simulink model "bh_source_XL_bigger"  (R2018a)
settings: Solver=ode4  StartTime=0.0  StopTime=60  FixedStep=0.001  RelTol=1e-5
model workspace (MAT data in the model file):
  Hz = 0.2
  L1x = 0.005
  L1y = 0.75
  L1z = 0.05
  L2x = 0.005
  L2y = 0.5
  L2z = 0.05
  L3x = 0.005
  L3y = 0.25
  L3z = 0.05
  P_mot.Vmax = 12
  P_mot.ID = 0
  P_mot.Ka = 0.04
  P_mot.Ke = 0.04
  P_mot.b = []
  P_mot.I = []
  P_mot.R = 5
  P_mot.L = 0.00063
  P_mot.G = 100
  P_mot.TQ_G_max = 3
  P_mot.TQ_m_max = 0.03
  Rturn = 0.05
  b1_damp = 0.005
  b2_damp = 0.005
  b3_damp = 0.005
  b4_damp = 0.005
  density = 1000
  g = 9.80665
  mass1 = 0.1875
  mass2 = 0.125
  mass3 = 0.0625
  mass4 = 1.57079632679
  theta1_0 = 0
  theta1_dot_0 = 0
  theta2_0 = 0
  theta2_dot_0 = 0
  theta3_0 = 0
  theta3_dot_0 = 0
  theta4_0 = 0
  theta4_dot_0 = 0
libraries: simulink_extras x2
settings Model: Creator=bhorton  LastModifiedBy=bhorton
settings SolverCC: ZeroCrossAlgorithm=Adaptive
settings OptimizationCC: LifeSpan=inf
settings DebuggingCC: SFUnexpectedBacktrackingDiag=warning  SFNoUnconditionalDefaultTransitionDiag=warning  SFExecutionAtInitializationDiag=none
settings CodeAppCC: StateflowObjectComments=on
settings GRTTargetCC: TargetLangStandard=C89/C90 (ANSI)
settings ConfigComp: CovMetricSettings=dw  CovHtmlReporting=on  CovSaveCumulativeToWorkspaceVar=on  CovSaveSingleToWorkspaceVar=on  CovExternalEMLEnable=off
settings SimscapeCC: SimscapeNormalizeSystem=off  SimscapeLogType=all  SimscapeLogDataHistory=10000  SelectedTab=Simscape Multibody
settings ExplorerConfigSet: InternalSimMechanicsExplorerSettings="<ExplorerConfiguration><canonicalview>default</canonicalview><AnimationSetting><BasePlaybackSpeed>1.0</BasePlaybackSpeed><PlaybackSpeedFactor>1.0</PlaybackSpeedFactor></AnimationSetting><TilePanel><TileInfo><Tiles Columns=\"2\" Count=\"4\" Rows=\"2\"><Column Left=\"2\" Weight=\"0.4992\"/><Column Left=\"655\" Weight=\"0.5008\"/><Column Left=\"1310\"/><Row Top=\"2\" Weight=\"0.4984\"/><Row Top=\"475\" Weight=\"0.5016\"/><Row Top=\"950\"/><Tile Height=\"1\" Width=\"1\" X=\"0\" Y=\"0\"/><Tile Height=\"1\" Width=\"1\" X=\"0\" Y=\"1\"/><Tile Height=\"1\" Width=\"1\" X=\"1\" Y=\"0\"/><Tile Height=\"1\" Width=\"1\" X=\"1\" Y=\"1\"/></Tiles></TileInfo><SceneInfo><SceneViewer><BGColor><R>0.60000002384185791</R><G>0.60000002384185791</G><B>0.60000002384185791</B></BGColor><Camera><DoPerspective>off</DoPerspective><Position><X>0.57010570867346566</X><Y>-0.81939487187068383</Y><Z>-0.041325690013103822</Z></Position><Center><X>0.57010570867346566</X><Y>0.37243777720020188</Y><Z>-0.041325690013103822</Z></Center><Up><X>0</X><Y>-0</Y><Z>1</Z></Up><ViewLimDist>1</ViewLimDist><YLim>0.58387397231837834</YLim><XLim>0.8103768064074045</XLim></Camera></SceneViewer><SceneViewer><BGColor><R>0.60000002384185791</R><G>0.60000002384185791</G><B>0.60000002384185791</B></BGColor><Camera><DoPerspective>off</DoPerspective><Position><X>0.51388092361444482</X><Y>0.52196280048326149</Y><Z>0.82022286793681332</Z></Position><Center><X>0.51388092361444482</X><Y>0.52196280048326149</Y><Z>-0.17977713206318668</Z></Center><Up><X>0</X><Y>1</Y><Z>-0</Z></Up><ViewLimDist>1</ViewLimDist><YLim>0.97737746692739225</YLim><XLim>1.3507104907751943</XLim></Camera></SceneViewer><SceneViewer><BGColor><R>0.60000002384185791</R><G>0.60000002384185791</G><B>0.60000002384185791</B></BGColor><Camera><DoPerspective>off</DoPerspective><Position><X>1.5094114010486579</X><Y>0.67796186035410533</Y><Z>-0.0082694811079057073</Z></Position><Center><X>0.47943838776152692</X><Y>0.67796186035410533</Y><Z>-0.0082694811079057073</Z></Center><Up><X>-0</X><Y>0</Y><Z>1</Z></Up><ViewLimDist>1</ViewLimDist><YLim>0.68608550995197048</YLim><XLim>0.95519663670037269</XLim></Camera></SceneViewer><SceneViewer><BGColor><R>0.60000002384185791</R><G>0.60000002384185791</G><B>0.60000002384185791</B></BGColor><Camera><DoPerspective>off</DoPerspective><Position><X>1.2860411296222924</X><Y>0.12259966358168611</Y><Z>0.94383913066063729</Z></Position><Center><X>0.57516484098717713</X><Y>0.83347595221680226</Y><Z>0.23296284202552392</Z></Center><Up><X>-0.40824829046386307</X><Y>0.40824829046386307</Y><Z>0.81649658092772615</Z></Up><ViewLimDist>1</ViewLimDist><YLim>0.94664886749230226</YLim><XLim>1.3123072283262387</XLim></Camera></SceneViewer></SceneInfo></TilePanel><MechEditorPanel><Cameras/><GfxPanelCameraMap/><VideoCreator><PlaybackSpeedRatio>1.0</PlaybackSpeedRatio><FrameRate>30</FrameRate><VideoFormat>Motion JPEG AVI</VideoFormat><FrameSize>auto</FrameSize></VideoCreator></MechEditorPanel></ExplorerConfiguration>"

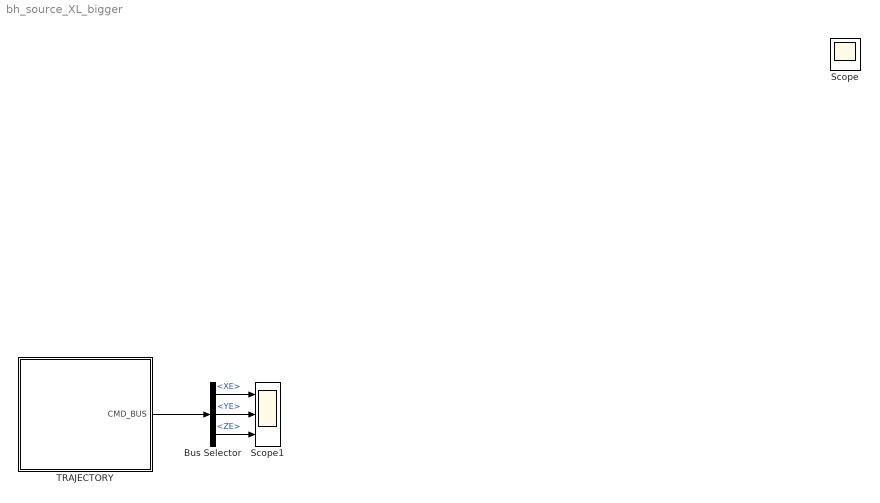
== system bh_source_XL_bigger ==
  Bus Selector : BusSelector  OutputSignals=XYZ_BUS.XE,XYZ_BUS.YE,XYZ_BUS.ZE
  Scope1 : Scope  NumInputPorts=3
  TRAJECTORY : Subsystem
  Scope : Scope
  wires:
  TRAJECTORY/1(CMD_BUS) -> Bus Selector/1
  Bus Selector/1 -> Scope1/1  "<XE>"
  Bus Selector/2 -> Scope1/2  "<YE>"
  Bus Selector/3 -> Scope1/3  "<ZE>"

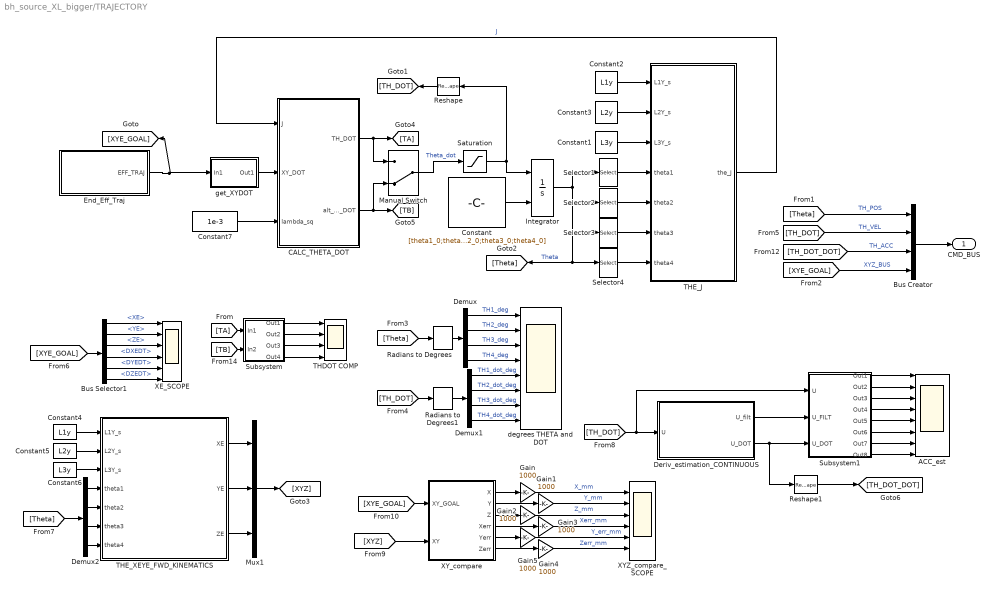
== system bh_source_XL_bigger/TRAJECTORY ==
  ACC_est : Scope  NumInputPorts=8
  Bus Creator : BusCreator  Inputs=4
  Bus Selector1 : BusSelector  OutputSignals=XE,YE,ZE,DXEDT,DYEDT,DZEDT
  CALC_THETA_DOT : MATLAB Function  TreatAsAtomicUnit=on
  Constant : Constant  Value=[theta1_0;theta2_0;theta3_0;theta4_0]  VectorParams1D=off
  Constant1 : Constant  Value=L3y
  Constant2 : Constant  Value=L1y
  Constant3 : Constant  Value=L2y
  Constant4 : Constant  Value=L1y
  Constant5 : Constant  Value=L2y
  Constant6 : Constant  Value=L3y
  Constant7 : Constant  Value=1e-3
  Demux : Demux
  Demux1 : Demux
  Demux2 : Demux
  Deriv_estimation_CONTINUOUS : Subsystem  mask(Derivative Estimation){wn=2*pi*100, p=1, x0_val=0, v0_val=0}
      mask prompts: wn "Natural frequency, wn (rad/sec)"; p "Damping ratio, p"; x0_val "X_IC"; v0_val "X_DOT_IC"
      mask help:
      | A simple derivative estimator using a 2nd order representation between input and output.
      |
      | The integrators use a discrete FORWARd Euler rule, and a sample time needs to be specified.
      mask init:
      | str0 = sprintf('fn = %.2f [Hz]', (wn/(2*pi)));
      | str1 = sprintf('wn = %.2f', wn);
      | str2 = sprintf('p  = %.3g', p);
      | %str3 = sprintf('dt = %.2g', dt);
      | str = char(str0,str1,str2);
      mask Display: disp(str)
  End_Eff_Traj : Subsystem
  Gain{,1..5} (6 alike) : Gain  Gain=1000
  Integrator : Integrator  InitialConditionSource=external
  Manual Switch : ManualSwitch  CurrentSetting=0
  Mux1 : Mux  Inputs=3
  Radians to Degrees : simulink_extras/Transformations/Radians to Degrees
  Radians to Degrees1 : simulink_extras/Transformations/Radians to Degrees
  Reshape : Reshape  OutputDimensionality=Column vector (2-D)
  Reshape1 : Reshape  OutputDimensionality=Column vector (2-D)
  Saturation : Saturate  UpperLimit=6  LowerLimit=-6
  Selector1 : Selector  InputPortWidth=4  IndexOptions=Index vector (dialog)  Indices=1  OutputSizes=1
  Selector2 : Selector  InputPortWidth=4  IndexOptions=Index vector (dialog)  Indices=2  OutputSizes=1
  Selector3 : Selector  InputPortWidth=4  IndexOptions=Index vector (dialog)  Indices=3  OutputSizes=1
  Selector4 : Selector  InputPortWidth=4  IndexOptions=Index vector (dialog)  Indices=4  OutputSizes=1
  Subsystem : Subsystem
  Subsystem1 : Subsystem
  THDOT COMP : Scope  NumInputPorts=4
  THE_J : MATLAB Function  TreatAsAtomicUnit=on
  THE_XEYE_FWD_KINEMATICS : MATLAB Function  TreatAsAtomicUnit=on
  XE_SCOPE : Scope  NumInputPorts=6
  XYZ_compare_SCOPE : Scope  NumInputPorts=6
  XY_compare : Subsystem
  degrees THETA and DOT : Scope  NumInputPorts=8
  get_XYDOT : Subsystem
  CMD_BUS : Outport
  wires:
  Bus Selector1/1 -> XE_SCOPE/1  "<XE>"
  Bus Selector1/2 -> XE_SCOPE/2  "<YE>"
  Bus Selector1/3 -> XE_SCOPE/3  "<ZE>"
  Bus Selector1/4 -> XE_SCOPE/4  "<DXEDT>"
  Bus Selector1/5 -> XE_SCOPE/5  "<DYEDT>"
  Bus Selector1/6 -> XE_SCOPE/6  "<DZEDT>"
  [XYE_GOAL] -> Bus Selector1/1
  Constant/1 -> Integrator/2
  THE_J/1(the_J) -> CALC_THETA_DOT/1(J)  "J"
  get_XYDOT/1(Out1) -> CALC_THETA_DOT/2(XY_DOT)
  Manual Switch/1 -> Saturation/1  "Theta_dot"
  Integrator/1 -> Selector4/1, [Theta], Selector3/1, Selector2/1, Selector1/1  "Theta"
  End_Eff_Traj/1(EFF_TRAJ) -> get_XYDOT/1(In1), [XYE_GOAL]
  Saturation/1 -> Integrator/1, Reshape/1
  Selector4/1 -> THE_J/7(theta4)
  Selector3/1 -> THE_J/6(theta3)
  Selector2/1 -> THE_J/5(theta2)
  Selector1/1 -> THE_J/4(theta1)
  Constant2/1 -> THE_J/1(L1Y_s)
  Constant3/1 -> THE_J/2(L2Y_s)
  Constant1/1 -> THE_J/3(L3Y_s)
  CALC_THETA_DOT/1(TH_DOT) -> [TA], Manual Switch/1
  CALC_THETA_DOT/2(alt_TH_DOT) -> [TB], Manual Switch/2
  Constant7/1 -> CALC_THETA_DOT/3(lambda_sq)
  [TB] -> Subsystem/2(In2)
  [TA] -> Subsystem/1(In1)
  Subsystem/1(Out1) -> THDOT COMP/1
  Subsystem/2(Out2) -> THDOT COMP/2
  Subsystem/3(Out3) -> THDOT COMP/3
  Subsystem/4(Out4) -> THDOT COMP/4
  [TH_DOT] -> Bus Creator/2  "TH_VEL"
  [Theta] -> Bus Creator/1  "TH_POS"
  Bus Creator/1 -> CMD_BUS/1
  Reshape/1 -> [TH_DOT]
  [XYE_GOAL] -> Bus Creator/4  "XYZ_BUS"
  Demux/4 -> degrees THETA and DOT/4  "TH4_deg"
  Demux/3 -> degrees THETA and DOT/3  "TH3_deg"
  Demux/2 -> degrees THETA and DOT/2  "TH2_deg"
  Demux/1 -> degrees THETA and DOT/1  "TH1_deg"
  Demux1/1 -> degrees THETA and DOT/5  "TH1_dot_deg"
  Demux1/2 -> degrees THETA and DOT/6  "TH2_dot_deg"
  Demux1/3 -> degrees THETA and DOT/7  "TH3_dot_deg"
  Demux1/4 -> degrees THETA and DOT/8  "TH4_dot_deg"
  [Theta] -> Radians to Degrees/1
  Radians to Degrees/1 -> Demux/1
  [TH_DOT] -> Radians to Degrees1/1
  Radians to Degrees1/1 -> Demux1/1
  Constant4/1 -> THE_XEYE_FWD_KINEMATICS/1(L1Y_s)
  Constant6/1 -> THE_XEYE_FWD_KINEMATICS/3(L3Y_s)
  Constant5/1 -> THE_XEYE_FWD_KINEMATICS/2(L2Y_s)
  Demux2/1 -> THE_XEYE_FWD_KINEMATICS/4(theta1)
  Demux2/2 -> THE_XEYE_FWD_KINEMATICS/5(theta2)
  Demux2/3 -> THE_XEYE_FWD_KINEMATICS/6(theta3)
  Demux2/4 -> THE_XEYE_FWD_KINEMATICS/7(theta4)
  [Theta] -> Demux2/1
  THE_XEYE_FWD_KINEMATICS/1(XE) -> Mux1/1
  THE_XEYE_FWD_KINEMATICS/3(ZE) -> Mux1/3
  THE_XEYE_FWD_KINEMATICS/2(YE) -> Mux1/2
  Mux1/1 -> [XYZ]
  [TH_DOT] -> Subsystem1/1(U), Deriv_estimation_CONTINUOUS/1(U)
  Subsystem1/1(Out1) -> ACC_est/1
  Subsystem1/2(Out2) -> ACC_est/2
  Subsystem1/3(Out3) -> ACC_est/3
  Subsystem1/4(Out4) -> ACC_est/4
  Subsystem1/5(Out5) -> ACC_est/5
  Subsystem1/6(Out6) -> ACC_est/6
  Subsystem1/7(Out7) -> ACC_est/7
  Subsystem1/8(Out8) -> ACC_est/8
  Deriv_estimation_CONTINUOUS/1(U_filt) -> Subsystem1/2(U_FILT)
  Deriv_estimation_CONTINUOUS/2(U_DOT) -> Reshape1/1, Subsystem1/3(U_DOT)
  [TH_DOT_DOT] -> Bus Creator/3  "TH_ACC"
  Reshape1/1 -> [TH_DOT_DOT]
  [XYZ] -> XY_compare/2(XY)
  [XYE_GOAL] -> XY_compare/1(XY_GOAL)
  Gain/1 -> XYZ_compare_SCOPE/1  "X_mm"
  Gain1/1 -> XYZ_compare_SCOPE/2  "Y_mm"
  Gain2/1 -> XYZ_compare_SCOPE/3  "Z_mm"
  XY_compare/1(X) -> Gain/1
  XY_compare/2(Y) -> Gain1/1
  XY_compare/3(Z) -> Gain2/1
  Gain4/1 -> XYZ_compare_SCOPE/6  "Zerr_mm"
  XY_compare/6(Zerr) -> Gain4/1
  XY_compare/5(Yerr) -> Gain5/1
  Gain5/1 -> XYZ_compare_SCOPE/5  "Y_err_mm"
  Gain3/1 -> XYZ_compare_SCOPE/4  "Xerr_mm"
  XY_compare/4(Xerr) -> Gain3/1

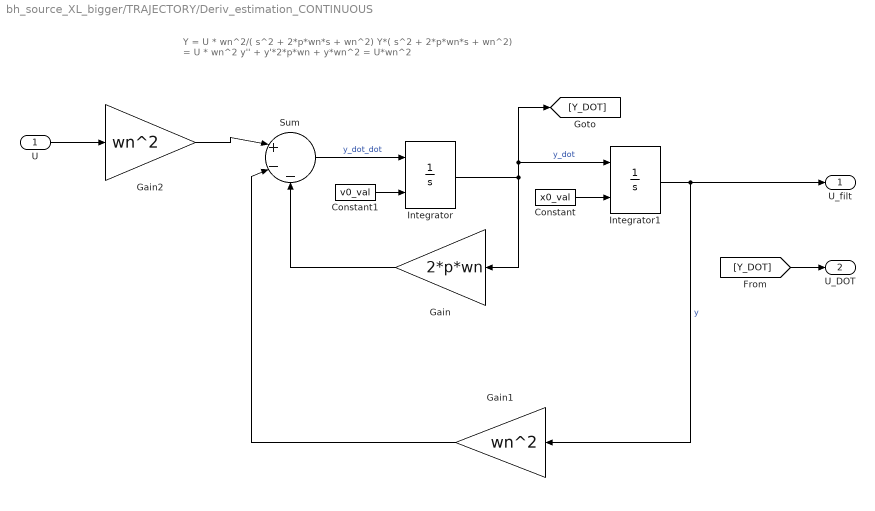
== system bh_source_XL_bigger/TRAJECTORY/Deriv_estimation_CONTINUOUS ==
  note: Y = U *     wn^2/( s^2 + 2*p*wn*s + wn^2)
      | Y*( s^2 + 2*p*wn*s + wn^2) = U * wn^2
      |
      | y'' + y'*2*p*wn + y*wn^2 = U*wn^2
  U : Inport
  Constant : Constant  Value=x0_val
  Constant1 : Constant  Value=v0_val
  Gain : Gain  Gain=2*p*wn
  Gain1 : Gain  Gain=wn^2
  Gain2 : Gain  Gain=wn^2
  Integrator : Integrator  InitialConditionSource=external
  Integrator1 : Integrator  InitialConditionSource=external
  Sum : Sum  Inputs=|+--
  U_filt : Outport
  U_DOT : Outport  Port=2
  wires:
  Integrator/1 -> Integrator1/1, [Y_DOT], Gain/1  "y_dot"
  Sum/1 -> Integrator/1  "y_dot_dot"
  Integrator1/1 -> U_filt/1, Gain1/1  "y"
  U/1 -> Gain2/1
  Gain2/1 -> Sum/1
  Gain/1 -> Sum/3
  Gain1/1 -> Sum/2
  [Y_DOT] -> U_DOT/1
  Constant/1 -> Integrator1/2
  Constant1/1 -> Integrator/2

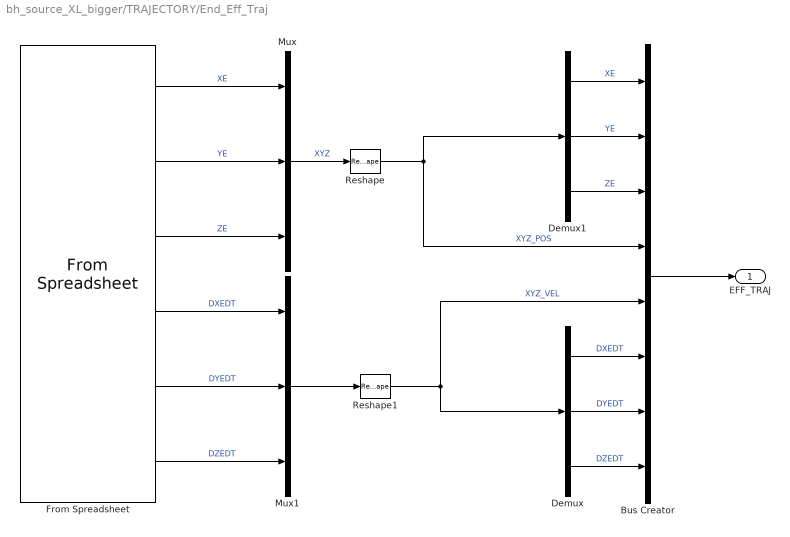
== system bh_source_XL_bigger/TRAJECTORY/End_Eff_Traj ==
  Bus Creator : BusCreator  Inputs=8
  Demux : Demux  Outputs=3
  Demux1 : Demux  Outputs=3
  From Spreadsheet : FromSpreadsheet  FileName=bh_hello_complete.xlsx  SheetName=COMP_SPLINE _4dof  SampleTime=0.001  ExtrapolationBeforeFirstDataPoint=Hold first value  ExtrapolationAfterLastDataPoint=Hold last value
  Mux : Mux  Inputs=3
  Mux1 : Mux  Inputs=3
  Reshape : Reshape  OutputDimensionality=Column vector (2-D)
  Reshape1 : Reshape  OutputDimensionality=Column vector (2-D)
  EFF_TRAJ : Outport
  wires:
  From Spreadsheet/2 -> Mux/2  "YE"
  From Spreadsheet/3 -> Mux/3  "ZE"
  From Spreadsheet/1 -> Mux/1  "XE"
  From Spreadsheet/4 -> Mux1/1  "DXEDT"
  Bus Creator/1 -> EFF_TRAJ/1
  From Spreadsheet/6 -> Mux1/3  "DZEDT"
  From Spreadsheet/5 -> Mux1/2  "DYEDT"
  Demux/1 -> Bus Creator/6  "DXEDT"
  Demux/2 -> Bus Creator/7  "DYEDT"
  Demux/3 -> Bus Creator/8  "DZEDT"
  Demux1/1 -> Bus Creator/1  "XE"
  Demux1/2 -> Bus Creator/2  "YE"
  Demux1/3 -> Bus Creator/3  "ZE"
  Mux/1 -> Reshape/1  "XYZ"
  Mux1/1 -> Reshape1/1
  Reshape/1 -> Bus Creator/4, Demux1/1  "XYZ_POS"
  Reshape1/1 -> Demux/1, Bus Creator/5  "XYZ_VEL"

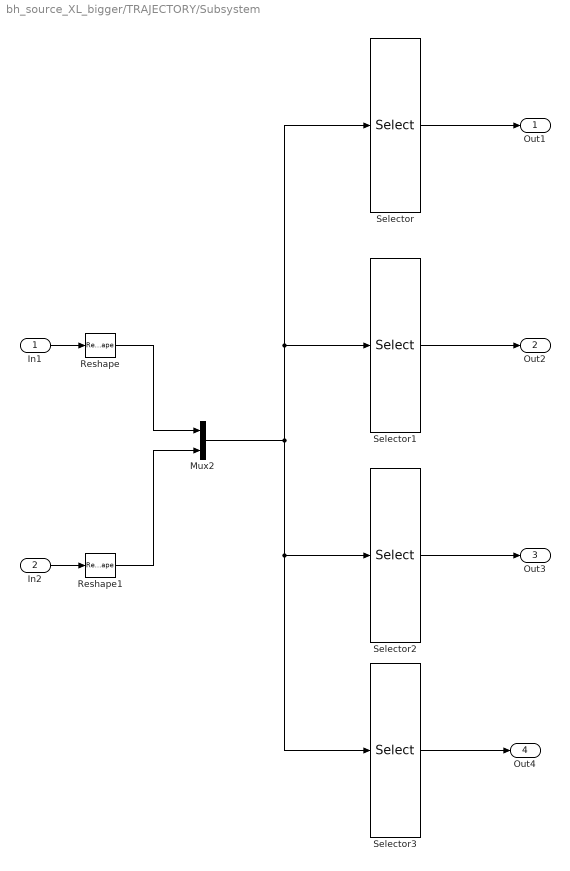
== system bh_source_XL_bigger/TRAJECTORY/Subsystem ==
  In1 : Inport
  In2 : Inport  Port=2
  Mux2 : Mux  Inputs=2
  Reshape : Reshape  OutputDimensionality=Column vector (2-D)
  Reshape1 : Reshape  OutputDimensionality=Column vector (2-D)
  Selector : Selector  InputPortWidth=8  IndexOptions=Index vector (dialog)  Indices=[1 5]  OutputSizes=1
  Selector1 : Selector  InputPortWidth=8  IndexOptions=Index vector (dialog)  Indices=[2 6]  OutputSizes=1
  Selector2 : Selector  InputPortWidth=8  IndexOptions=Index vector (dialog)  Indices=[3 7]  OutputSizes=1
  Selector3 : Selector  InputPortWidth=8  IndexOptions=Index vector (dialog)  Indices=[4 8]  OutputSizes=1
  Out1 : Outport
  Out2 : Outport  Port=2
  Out3 : Outport  Port=3
  Out4 : Outport  Port=4
  wires:
  In1/1 -> Reshape/1
  In2/1 -> Reshape1/1
  Reshape/1 -> Mux2/1
  Reshape1/1 -> Mux2/2
  Selector2/1 -> Out3/1
  Selector1/1 -> Out2/1
  Selector/1 -> Out1/1
  Mux2/1 -> Selector1/1, Selector/1, Selector2/1, Selector3/1
  Selector3/1 -> Out4/1

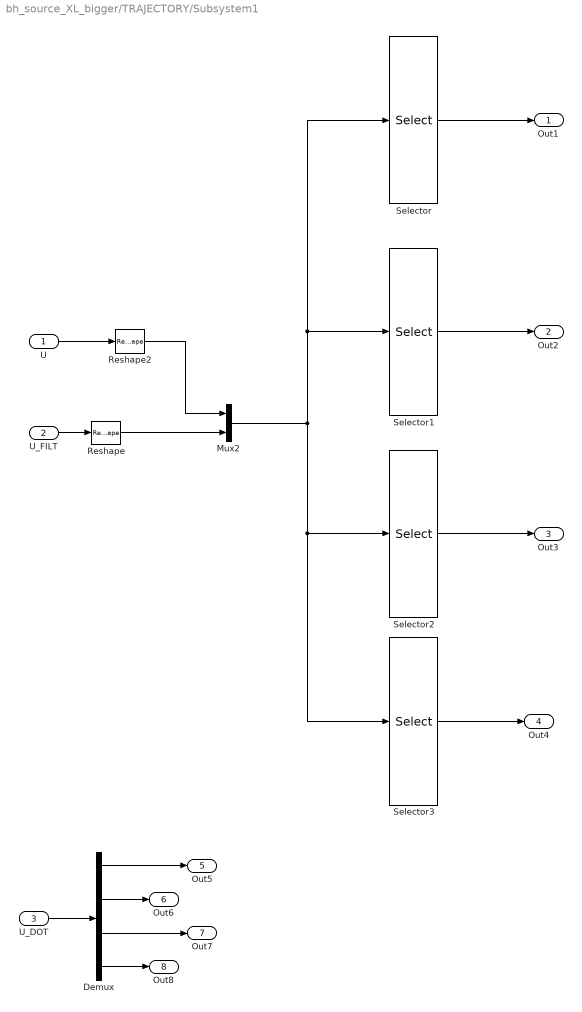
== system bh_source_XL_bigger/TRAJECTORY/Subsystem1 ==
  U : Inport
  U_FILT : Inport  Port=2
  U_DOT : Inport  Port=3
  Demux : Demux
  Mux2 : Mux  Inputs=2
  Reshape : Reshape  OutputDimensionality=Column vector (2-D)
  Reshape2 : Reshape  OutputDimensionality=Column vector (2-D)
  Selector : Selector  InputPortWidth=8  IndexOptions=Index vector (dialog)  Indices=[1 5]  OutputSizes=1
  Selector1 : Selector  InputPortWidth=8  IndexOptions=Index vector (dialog)  Indices=[2 6]  OutputSizes=1
  Selector2 : Selector  InputPortWidth=8  IndexOptions=Index vector (dialog)  Indices=[3 7]  OutputSizes=1
  Selector3 : Selector  InputPortWidth=8  IndexOptions=Index vector (dialog)  Indices=[4 8]  OutputSizes=1
  Out1 : Outport
  Out2 : Outport  Port=2
  Out3 : Outport  Port=3
  Out4 : Outport  Port=4
  Out5 : Outport  Port=5
  Out6 : Outport  Port=6
  Out7 : Outport  Port=7
  Out8 : Outport  Port=8
  wires:
  U_FILT/1 -> Reshape/1
  U_DOT/1 -> Demux/1
  Selector2/1 -> Out3/1
  Selector1/1 -> Out2/1
  Selector/1 -> Out1/1
  Mux2/1 -> Selector1/1, Selector/1, Selector2/1, Selector3/1
  Selector3/1 -> Out4/1
  U/1 -> Reshape2/1
  Reshape/1 -> Mux2/2
  Reshape2/1 -> Mux2/1
  Demux/1 -> Out5/1
  Demux/2 -> Out6/1
  Demux/3 -> Out7/1
  Demux/4 -> Out8/1

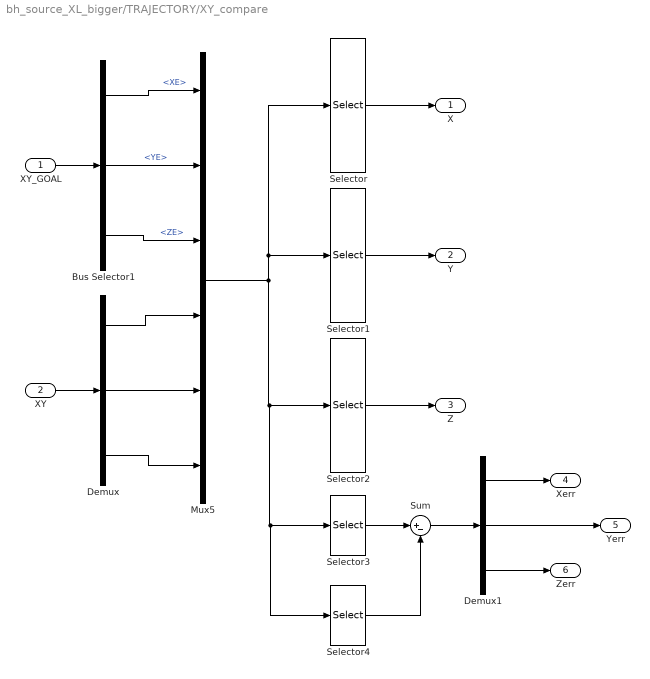
== system bh_source_XL_bigger/TRAJECTORY/XY_compare ==
  XY_GOAL : Inport
  XY : Inport  Port=2
  Bus Selector1 : BusSelector  OutputSignals=XE,YE,ZE
  Demux : Demux  Outputs=3
  Demux1 : Demux  Outputs=3
  Mux5 : Mux  Inputs=6
  Selector : Selector  InputPortWidth=6  IndexOptions=Index vector (dialog)  Indices=[1 4]  OutputSizes=1
  Selector1 : Selector  InputPortWidth=6  IndexOptions=Index vector (dialog)  Indices=[2 5]  OutputSizes=1
  Selector2 : Selector  InputPortWidth=6  IndexOptions=Index vector (dialog)  Indices=[3 6]  OutputSizes=1
  Selector3 : Selector  InputPortWidth=6  IndexOptions=Index vector (dialog)  Indices=[1 2 3]  OutputSizes=1
  Selector4 : Selector  InputPortWidth=6  IndexOptions=Index vector (dialog)  Indices=[4 5 6]  OutputSizes=1
  Sum : Sum  Inputs=|+-
  X : Outport
  Y : Outport  Port=2
  Z : Outport  Port=3
  Xerr : Outport  Port=4
  Yerr : Outport  Port=5
  Zerr : Outport  Port=6
  wires:
  XY_GOAL/1 -> Bus Selector1/1
  XY/1 -> Demux/1
  Bus Selector1/3 -> Mux5/3  "<ZE>"
  Bus Selector1/2 -> Mux5/2  "<YE>"
  Bus Selector1/1 -> Mux5/1  "<XE>"
  Demux/1 -> Mux5/4
  Demux/2 -> Mux5/5
  Demux/3 -> Mux5/6
  Mux5/1 -> Selector4/1, Selector3/1, Selector2/1, Selector1/1, Selector/1
  Selector2/1 -> Z/1
  Selector/1 -> X/1
  Selector1/1 -> Y/1
  Selector3/1 -> Sum/1
  Selector4/1 -> Sum/2
  Sum/1 -> Demux1/1
  Demux1/1 -> Xerr/1
  Demux1/2 -> Yerr/1
  Demux1/3 -> Zerr/1

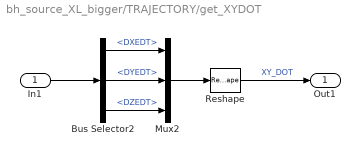
== system bh_source_XL_bigger/TRAJECTORY/get_XYDOT ==
  In1 : Inport
  Bus Selector2 : BusSelector  OutputSignals=DXEDT,DYEDT,DZEDT
  Mux2 : Mux  Inputs=3
  Reshape : Reshape  OutputDimensionality=Column vector (2-D)
  Out1 : Outport
  wires:
  Bus Selector2/1 -> Mux2/1  "<DXEDT>"
  Bus Selector2/2 -> Mux2/2  "<DYEDT>"
  In1/1 -> Bus Selector2/1
  Mux2/1 -> Reshape/1
  Reshape/1 -> Out1/1  "XY_DOT"
  Bus Selector2/3 -> Mux2/3  "<DZEDT>"

== matlab function bh_source_XL_bigger/TRAJECTORY/THE_J ==
  data: L1Y_s input; the_J output; L2Y_s input; L3Y_s input; theta1 input; theta2 input; theta3 input; theta4 input
function the_J = THE_J(L1Y_s,L2Y_s,L3Y_s,theta1,theta2,theta3,theta4)
%#codegen

%    This function was generated by the Symbolic Math Toolbox version 7.0.
%    13-Sep-2016 14:49:06

the_J = reshape([sin(theta4).*(L2Y_s.*sin(theta1+theta2)+L1Y_s.*sin(theta1)+L3Y_s.*sin(theta1+theta2+theta3)),-cos(theta4).*(L2Y_s.*sin(theta1+theta2)+L1Y_s.*sin(theta1)+L3Y_s.*sin(theta1+theta2+theta3)),L2Y_s.*cos(theta1+theta2)+L1Y_s.*cos(theta1)+L3Y_s.*cos(theta1+theta2+theta3),sin(theta4).*(L2Y_s.*sin(theta1+theta2)+L3Y_s.*sin(theta1+theta2+theta3)),-cos(theta4).*(L2Y_s.*sin(theta1+theta2)+L3Y_s.*sin(theta1+theta2+theta3)),L2Y_s.*cos(theta1+theta2)+L3Y_s.*cos(theta1+theta2+theta3),L3Y_s.*sin(theta1+theta2+theta3).*sin(theta4),-L3Y_s.*sin(theta1+theta2+theta3).*cos(theta4),L3Y_s.*cos(theta1+theta2+theta3),-cos(theta4).*(L2Y_s.*cos(theta1+theta2)+L1Y_s.*cos(theta1)+L3Y_s.*cos(theta1+theta2+theta3)),-sin(theta4).*(L2Y_s.*cos(theta1+theta2)+L1Y_s.*cos(theta1)+L3Y_s.*cos(theta1+theta2+theta3)),0.0],[3,4]);

== matlab function bh_source_XL_bigger/TRAJECTORY/CALC_THETA_DOT ==
  data: J input; TH_DOT output; XY_DOT input; lambda_sq input; alt_TH_DOT output
function [TH_DOT, alt_TH_DOT] = calc_TH_DOT(J, XY_DOT, lambda_sq)
%#codegen

    %% so our problem is this:
    %     J*q_dot = x_dot
    %
    % so a solution is:
    %
    %      q_dot = pinv(J) * x_dot
    
    TH_DOT = pinv(J) * XY_DOT;

    %% we can also penalise the q_dot by applying a weight to it.
    %  this will give us a solution where we get a "smaller" q_dot.  This
    %  acts as a "dampening" agent ... and we notice it most at startup.
    
    % consider solving the REGULARISED problem
    %     [       J_mxn  ] * q_dot =  [ x_dot ]
    %     [lamb^2*I_nxn  ]            [ 0_nx1 ]
    %
    % which we'll wite as:
    %
    %              new_A * q_dot = new_b
    %
    % so a solution is:
    %
    %      q_dot = pinv(new_A) * new_b
    
    [m, n]     = size(J); 
    I_mat      = eye( n ); 
    new_A      = [ J;
                   lambda_sq * I_mat];

    new_b      = [ XY_DOT;
                   zeros(n,1) ];

    alt_TH_DOT = pinv( new_A  ) * new_b;
end

== matlab function bh_source_XL_bigger/TRAJECTORY/THE_XEYE_FWD_KINEMATICS ==
  data: L1Y_s input; XE output; L2Y_s input; L3Y_s input; theta1 input; theta2 input; theta3 input; theta4 input; YE output; ZE output
function [XE,YE,ZE] = THE_XEYE(L1Y_s,L2Y_s,L3Y_s,theta1,theta2,theta3,theta4)
%#codegen

%    This function was generated by the Symbolic Math Toolbox version 7.0.
%    13-Sep-2016 15:29:58

XE = -sin(theta4).*(L2Y_s.*cos(theta1+theta2)+L1Y_s.*cos(theta1)+L3Y_s.*cos(theta1+theta2+theta3));
if nargout > 1
    YE = cos(theta4).*(L2Y_s.*cos(theta1+theta2)+L1Y_s.*cos(theta1)+L3Y_s.*cos(theta1+theta2+theta3));
end
if nargout > 2
    ZE = L2Y_s.*sin(theta1+theta2)+L1Y_s.*sin(theta1)+L3Y_s.*sin(theta1+theta2+theta3);
end
